simulink model "APP_VD"  (R2018a)
settings: configuration reference "cs_ert" (kept outside this file)
model workspace (MAT data in the model file):
  APP_VD_DT = 10
values from neighbouring files (symbols this model uses):
  APP_drLinRmp_C = 5.0    [APP_VD.sldd]
  APP_facLowNegPT1_C = 50.0    [APP_VD.sldd]
  APP_facLowPosPT1_C = 50.0    [APP_VD.sldd]
  APP_facMidNegPT1_C = 50.0    [APP_VD.sldd]
  APP_facMidPosPT1_C = 50.0    [APP_VD.sldd]
  APP_facUppNegPT1_C = 50.0    [APP_VD.sldd]
  APP_facUppPosPT1_C = 50.0    [APP_VD.sldd]
  APP_rThrFltLowNeg_C = 25.0    [APP_VD.sldd]
  APP_rThrFltLowPos_C = 25.0    [APP_VD.sldd]
  APP_rThrFltMidNeg_C = 50.0    [APP_VD.sldd]
  APP_rThrFltMidPos_C = 50.0    [APP_VD.sldd]
  APP_swtEnaFlt_C = 0    [APP_VD.sldd]
  APP_swtEnaUnJit_C = 0    [APP_VD.sldd]
  APP_uJitter_C = 3.0    [APP_VD.sldd]
  MoFAPP_rLinAPPCURCalMsgA_CUR : value not decoded    [APP_VD.sldd]
  MoFAPP_rLinAPPCURCalMsgA_CURX : value not decoded    [APP_VD.sldd]
  SigTst_rAPP_C = 0.0    [APP_VD.sldd]
  SigTst_swtAPP_C = 0    [APP_VD.sldd]
undefined symbols (not defined in the file or in its folder): Switch
libraries: sllib x2, simulink x1
settings Model: DataDictionary=APP_VD.sldd  Creator=zhoutinglin  LastModifiedBy=zhoutinglin

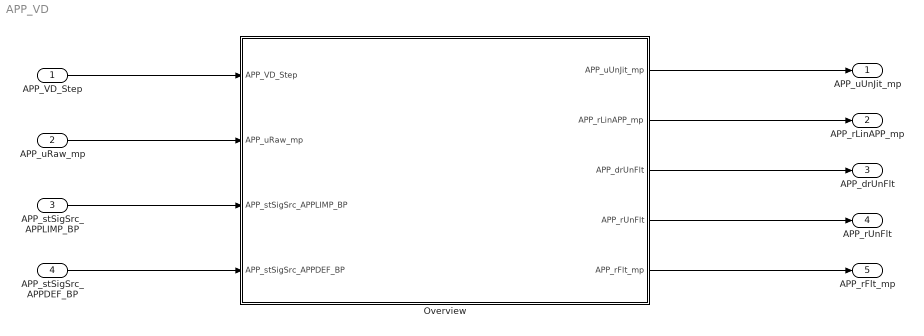
== system APP_VD ==
  APP_VD_Step : Inport  OutputFunctionCall=on
  APP_uRaw_mp : Inport  Description=Acceleration pedal position raw value  Port=2  OutMin=0  OutMax=5000  OutDataTypeStr=Volt_mV  Unit=mv  PortDimensions=[1 1]
  APP_stSigSrc_APPLIMP_BP : Inport  Description=Substitute operation active, accelerator pedal sensor value and accelerator pedal sensor increase are limited  Port=3  OutMin=0  OutMax=1  OutDataTypeStr=boolean  PortDimensions=[1 1]
  APP_stSigSrc_APPDEF_BP : Inport  Description=both the sensors are defective. Use the default value  Port=4  OutMin=0  OutMax=1  OutDataTypeStr=boolean  PortDimensions=[1 1]
  Overview : Subsystem
  APP_uUnJit_mp : Outport  Description=Acceleration pedal position unjittered value  OutMin=0  OutMax=5000  OutDataTypeStr=Volt_mV  Unit=mv  PortDimensions=[1 1]
  APP_rLinAPP_mp : Outport  Description=Linearisation ratio of accelerator pedal  Port=2  OutMin=0  OutMax=100  OutDataTypeStr=Percent  Unit=%  PortDimensions=[1 1]
  APP_drUnFlt : Outport  Description=Acceleration pedal position gradient of unfilterd value  Port=3  OutMin=-200  OutMax=200  OutDataTypeStr=Percent_s  Unit=%/ms  PortDimensions=[1 1]
  APP_rUnFlt : Outport  Description=Unfiltered APP value  Port=4  OutMin=0  OutMax=100  OutDataTypeStr=Percent  Unit=%  PortDimensions=[1 1]
  APP_rFlt_mp : Outport  Description=Acceleration pedal position filtered value  Port=5  OutMin=0  OutMax=100  OutDataTypeStr=Percent  Unit=%  PortDimensions=[1 1]
  wires:
  APP_VD_Step/1 -> Overview/1(APP_VD_Step)
  APP_uRaw_mp/1 -> Overview/2(APP_uRaw_mp)
  APP_stSigSrc_APPLIMP_BP/1 -> Overview/3(APP_stSigSrc_APPLIMP_BP)
  APP_stSigSrc_APPDEF_BP/1 -> Overview/4(APP_stSigSrc_APPDEF_BP)
  Overview/1(APP_uUnJit_mp) -> APP_uUnJit_mp/1
  Overview/2(APP_rLinAPP_mp) -> APP_rLinAPP_mp/1
  Overview/3(APP_drUnFlt) -> APP_drUnFlt/1
  Overview/4(APP_rUnFlt) -> APP_rUnFlt/1
  Overview/5(APP_rFlt_mp) -> APP_rFlt_mp/1

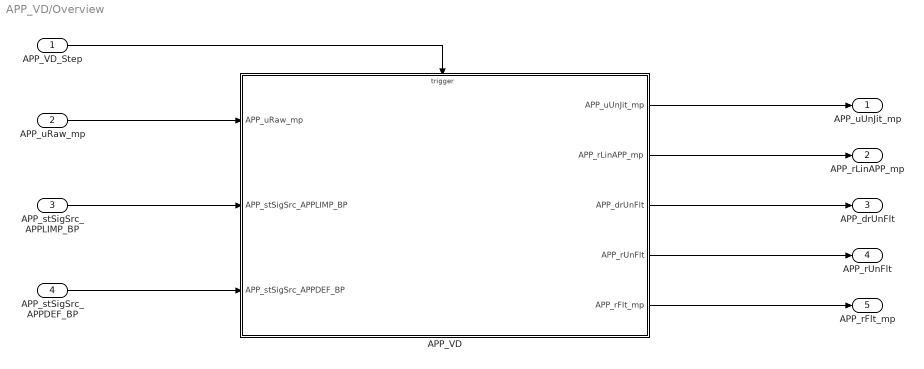
== system APP_VD/Overview ==
  APP_VD_Step : Inport
  APP_uRaw_mp : Inport  Port=2
  APP_stSigSrc_APPLIMP_BP : Inport  Port=3
  APP_stSigSrc_APPDEF_BP : Inport  Port=4
  APP_VD : Subsystem
  APP_uUnJit_mp : Outport
  APP_rLinAPP_mp : Outport  Port=2
  APP_drUnFlt : Outport  Port=3
  APP_rUnFlt : Outport  Port=4
  APP_rFlt_mp : Outport  Port=5
  wires:
  APP_uRaw_mp/1 -> APP_VD/1(APP_uRaw_mp)
  APP_stSigSrc_APPLIMP_BP/1 -> APP_VD/2(APP_stSigSrc_APPLIMP_BP)
  APP_stSigSrc_APPDEF_BP/1 -> APP_VD/3(APP_stSigSrc_APPDEF_BP)
  APP_VD/1(APP_uUnJit_mp) -> APP_uUnJit_mp/1
  APP_VD/2(APP_rLinAPP_mp) -> APP_rLinAPP_mp/1
  APP_VD/3(APP_drUnFlt) -> APP_drUnFlt/1
  APP_VD/4(APP_rUnFlt) -> APP_rUnFlt/1
  APP_VD/5(APP_rFlt_mp) -> APP_rFlt_mp/1
  APP_VD_Step/1 -> APP_VD/Trigger

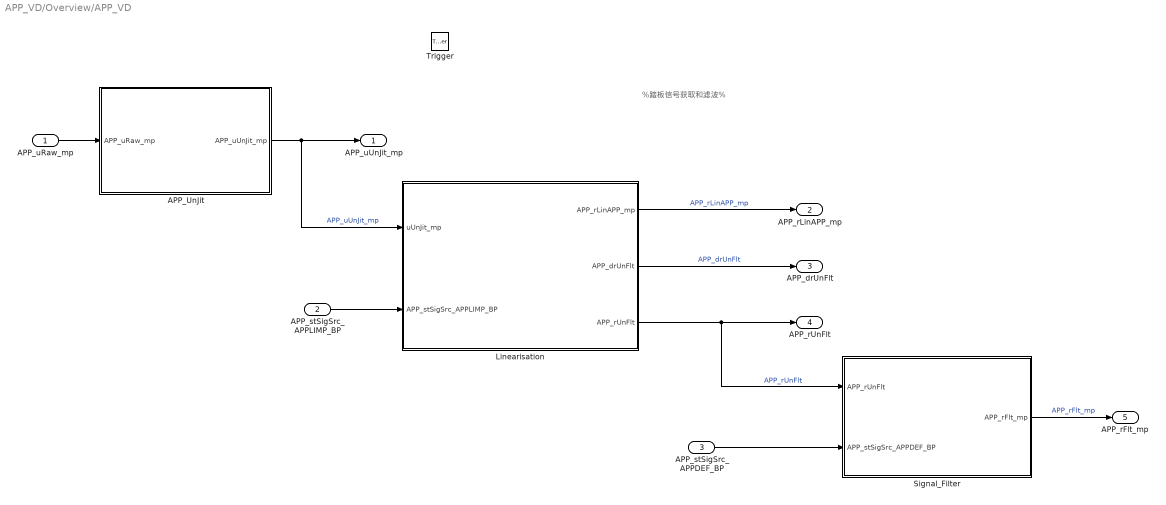
== system APP_VD/Overview/APP_VD ==
  note: %踏板信号获取和滤波%
  APP_uRaw_mp : Inport  Tag=mv
  APP_stSigSrc_APPLIMP_BP : Inport  Port=2
  APP_stSigSrc_APPDEF_BP : Inport  Port=3
  Trigger : TriggerPort  TriggerType=function-call  VariantControl=Variant  PortDimensions=1
  APP_UnJit : Subsystem
  Linearisation : Subsystem
  Signal_Filter : Subsystem
  APP_uUnJit_mp : Outport  Tag=mv
  APP_rLinAPP_mp : Outport  Tag=%  Port=2
  APP_drUnFlt : Outport  Tag=%/s  Port=3
  APP_rUnFlt : Outport  Tag=%  Port=4
  APP_rFlt_mp : Outport  Tag=%  Port=5
  wires:
  APP_uRaw_mp/1 -> APP_UnJit/1(APP_uRaw_mp)
  Signal_Filter/1(APP_rFlt_mp) -> APP_rFlt_mp/1  "APP_rFlt_mp"
  Linearisation/2(APP_drUnFlt) -> APP_drUnFlt/1  "APP_drUnFlt"
  APP_stSigSrc_APPDEF_BP/1 -> Signal_Filter/2(APP_stSigSrc_APPDEF_BP)
  Linearisation/3(APP_rUnFlt) -> APP_rUnFlt/1, Signal_Filter/1(APP_rUnFlt)  "APP_rUnFlt"
  Linearisation/1(APP_rLinAPP_mp) -> APP_rLinAPP_mp/1  "APP_rLinAPP_mp"
  APP_stSigSrc_APPLIMP_BP/1 -> Linearisation/2(APP_stSigSrc_APPLIMP_BP)
  APP_UnJit/1(APP_uUnJit_mp) -> APP_uUnJit_mp/1, Linearisation/1(uUnJit_mp)  "APP_uUnJit_mp"

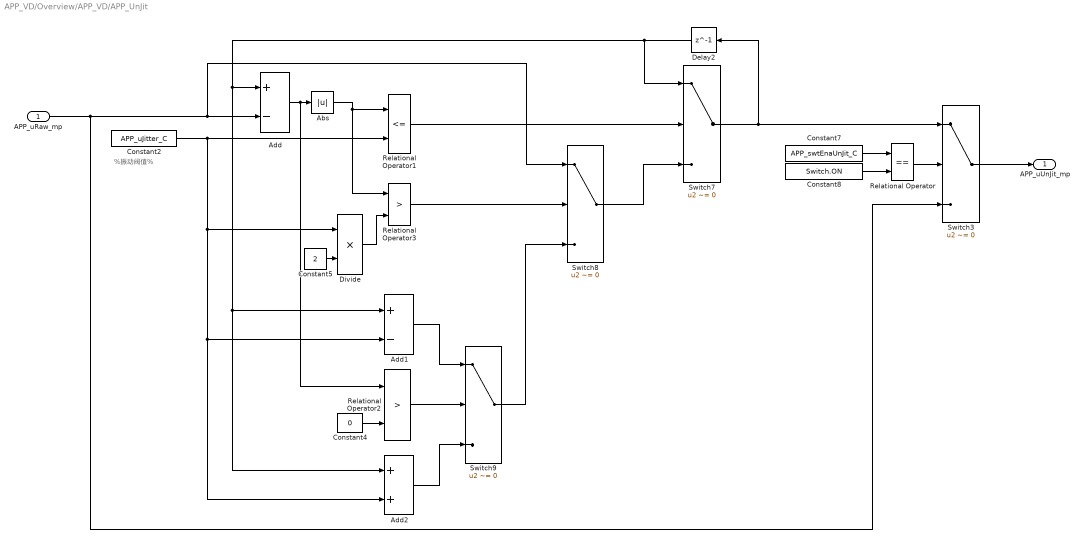
== system APP_VD/Overview/APP_VD/APP_UnJit ==
  note: %振动阀值%
  APP_uRaw_mp : Inport
  Abs : Abs  OutDataTypeStr=Inherit: Inherit via back propagation
  Add : Sum  Inputs=+-  InputSameDT=on
  Add1 : Sum  Inputs=+-  InputSameDT=on
  Add2 : Sum  InputSameDT=on
  Constant2 : Constant  Value=APP_uJitter_C
  Constant4 : Constant  Value=0  OutDataTypeStr=Inherit: Inherit via back propagation
  Constant5 : Constant  Value=2  OutDataTypeStr=Inherit: Inherit via back propagation
  Constant7 : Constant  Value=APP_swtEnaUnJit_C
  Constant8 : Constant  Value=Switch.ON  OutDataTypeStr=Inherit: Inherit via back propagation
  Delay2 : Delay  DelayLength=1  InitialCondition=0
  Divide : Product  Inputs=**  OutDataTypeStr=Inherit: Inherit via back propagation
  Relational Operator : RelationalOperator  Operator===  OutDataTypeStr=boolean  RndMeth=Simplest  InputSameDT=on
  Relational Operator1 : RelationalOperator  Operator=<=  OutDataTypeStr=boolean  RndMeth=Nearest  InputSameDT=on
  Relational Operator2 : RelationalOperator  Operator=>  OutDataTypeStr=boolean  RndMeth=Nearest  InputSameDT=on
  Relational Operator3 : RelationalOperator  Operator=>  OutDataTypeStr=boolean  RndMeth=Nearest  InputSameDT=on
  Switch{3,7..9} (4 alike) : Switch  Criteria=u2 ~= 0  InputSameDT=on
  APP_uUnJit_mp : Outport
  wires:
  Constant2/1 -> Add2/2, Add1/2, Divide/1, Relational Operator1/2
  Relational Operator/1 -> Switch3/2
  Add1/1 -> Switch9/1
  Add2/1 -> Switch9/3
  Add/1 -> Abs/1, Relational Operator2/1
  Abs/1 -> Relational Operator1/1, Relational Operator3/1
  Constant8/1 -> Relational Operator/2
  Switch9/1 -> Switch8/3
  Divide/1 -> Relational Operator3/2
  Relational Operator1/1 -> Switch7/2
  Relational Operator3/1 -> Switch8/2
  Delay2/1 -> Add1/1, Add2/1, Add/1, Switch7/1
  Switch7/1 -> Switch3/1, Delay2/1
  Constant5/1 -> Divide/2
  APP_uRaw_mp/1 -> Switch3/3, Add/2, Switch8/1
  Relational Operator2/1 -> Switch9/2
  Constant4/1 -> Relational Operator2/2
  Switch8/1 -> Switch7/3
  Constant7/1 -> Relational Operator/1
  Switch3/1 -> APP_uUnJit_mp/1

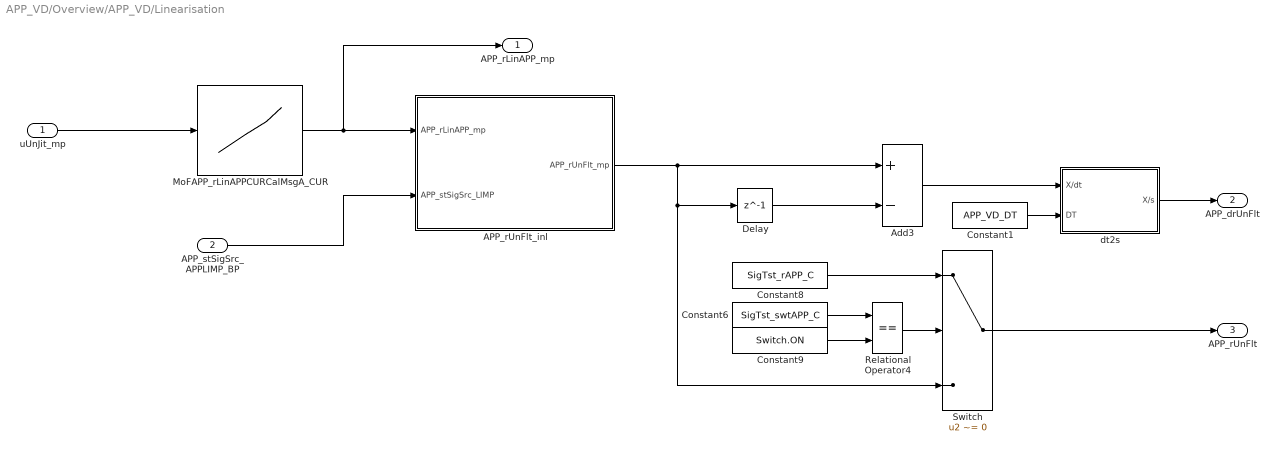
== system APP_VD/Overview/APP_VD/Linearisation ==
  uUnJit_mp : Inport
  APP_stSigSrc_APPLIMP_BP : Inport  Tag=-  Port=2
  APP_rUnFlt_inl : Subsystem
  Add3 : Sum  Inputs=+-  InputSameDT=on
  Constant1 : Constant  Value=APP_VD_DT  OutDataTypeStr=Inherit: Inherit via back propagation
  Constant6 : Constant  Value=SigTst_swtAPP_C
  Constant8 : Constant  Value=SigTst_rAPP_C
  Constant9 : Constant  Value=Switch.ON  OutDataTypeStr=Inherit: Inherit via back propagation
  Delay : Delay  DelayLength=1  InitialCondition=0
  MoFAPP_rLinAPPCURCalMsgA_CUR : Lookup_n-D  NumberOfTableDimensions=1  BreakpointsForDimension1=MoFAPP_rLinAPPCURCalMsgA_CURX  IndexSearchMethod=Linear search  BeginIndexSearchUsingPreviousIndexResult=on  UseOneInputPortForAllInputData=on  Table=MoFAPP_rLinAPPCURCalMsgA_CUR  ExtrapMethod=Clip  UseLastTableValue=on  InternalRulePriority=Speed  OutDataTypeStr=Inherit: Inherit via back propagation  SaturateOnIntegerOverflow=on
  Relational Operator4 : RelationalOperator  Operator===  OutDataTypeStr=boolean  RndMeth=Simplest  InputSameDT=on
  Switch : Switch  Criteria=u2 ~= 0  InputSameDT=on
  dt2s : Subsystem
  APP_rLinAPP_mp : Outport  Tag=%%
  APP_drUnFlt : Outport  Tag=%%  Port=2
  APP_rUnFlt : Outport  Tag=%%  Port=3
  wires:
  APP_stSigSrc_APPLIMP_BP/1 -> APP_rUnFlt_inl/2(APP_stSigSrc_LIMP)
  uUnJit_mp/1 -> MoFAPP_rLinAPPCURCalMsgA_CUR/1
  Relational Operator4/1 -> Switch/2
  Constant6/1 -> Relational Operator4/1
  Constant9/1 -> Relational Operator4/2
  Constant8/1 -> Switch/1
  Switch/1 -> APP_rUnFlt/1
  Delay/1 -> Add3/2
  APP_rUnFlt_inl/1(APP_rUnFlt_mp) -> Switch/3, Delay/1, Add3/1
  MoFAPP_rLinAPPCURCalMsgA_CUR/1 -> APP_rLinAPP_mp/1, APP_rUnFlt_inl/1(APP_rLinAPP_mp)
  Constant1/1 -> dt2s/2(DT)
  Add3/1 -> dt2s/1(X/dt)
  dt2s/1(X/s) -> APP_drUnFlt/1

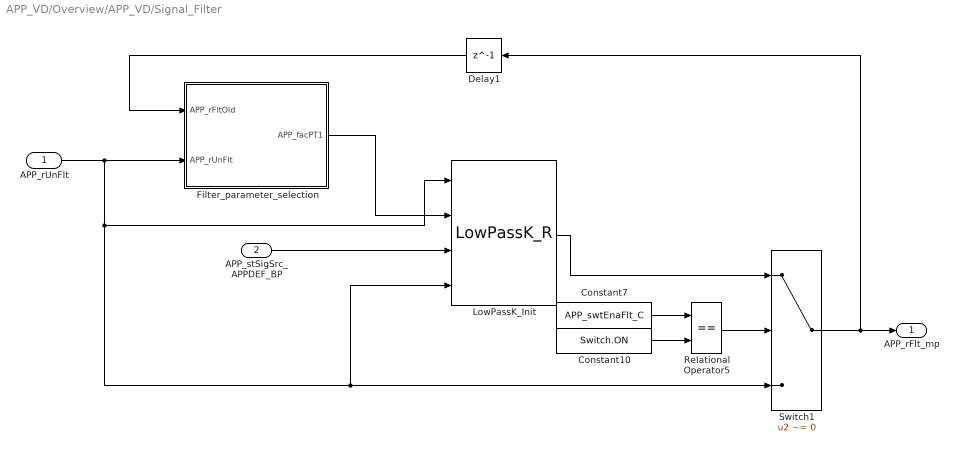
== system APP_VD/Overview/APP_VD/Signal_Filter ==
  APP_rUnFlt : Inport
  APP_stSigSrc_APPDEF_BP : Inport  Tag=-  Port=2
  Constant10 : Constant  Value=Switch.ON  OutDataTypeStr=Inherit: Inherit via back propagation
  Constant7 : Constant  Value=APP_swtEnaFlt_C
  Delay1 : Delay  DelayLength=1  InitialCondition=0
  Filter_parameter_selection : Subsystem  TreatAsAtomicUnit=on
  LowPassK_Init : sllib/LowPassK_R
      settings: SourceProductName=sllib
  Relational Operator5 : RelationalOperator  Operator===  OutDataTypeStr=boolean  RndMeth=Simplest  InputSameDT=on
  Switch1 : Switch  Criteria=u2 ~= 0  InputSameDT=on
  APP_rFlt_mp : Outport  Tag=%%
  wires:
  Relational Operator5/1 -> Switch1/2
  Constant10/1 -> Relational Operator5/2
  Constant7/1 -> Relational Operator5/1
  LowPassK_Init/1 -> Switch1/1
  Filter_parameter_selection/1(APP_facPT1) -> LowPassK_Init/2
  Switch1/1 -> APP_rFlt_mp/1, Delay1/1
  Delay1/1 -> Filter_parameter_selection/1(APP_rFltOld)
  APP_rUnFlt/1 -> LowPassK_Init/4, Switch1/3, LowPassK_Init/1, Filter_parameter_selection/2(APP_rUnFlt)
  APP_stSigSrc_APPDEF_BP/1 -> LowPassK_Init/3

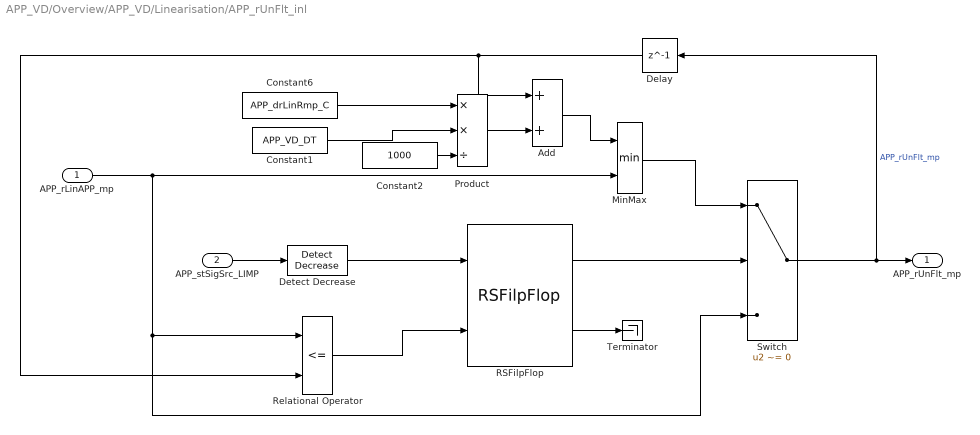
== system APP_VD/Overview/APP_VD/Linearisation/APP_rUnFlt_inl ==
  APP_rLinAPP_mp : Inport
  APP_stSigSrc_LIMP : Inport  Port=2
  Add : Sum  InputSameDT=on
  Constant1 : Constant  Value=APP_VD_DT  OutDataTypeStr=Inherit: Inherit via back propagation
  Constant2 : Constant  Value=1000  OutDataTypeStr=int16
  Constant6 : Constant  Value=APP_drLinRmp_C
  Delay : Delay  DelayLength=1  InitialCondition=0
  Detect Decrease : simulink/Logic and Bit Operations/Detect Decrease  vinit=0.0  OutDataTypeStr=boolean
  MinMax : MinMax  Inputs=2
  Product : Product  Inputs=**/  OutDataTypeStr=Inherit: Inherit via back propagation
  RSFilpFlop : sllib/RSFilpFlop
      settings: SourceProductName=sllib
  Relational Operator : RelationalOperator  Operator=<=  OutDataTypeStr=boolean  RndMeth=Simplest
  Switch : Switch  Criteria=u2 ~= 0  InputSameDT=on
  Terminator : Terminator
  APP_rUnFlt_mp : Outport
  wires:
  RSFilpFlop/2 -> Terminator/1
  Relational Operator/1 -> RSFilpFlop/2
  APP_stSigSrc_LIMP/1 -> Detect Decrease/1
  Detect Decrease/1 -> RSFilpFlop/1
  Delay/1 -> Relational Operator/2, Add/1
  Switch/1 -> APP_rUnFlt_mp/1, Delay/1  "APP_rUnFlt_mp"
  Add/1 -> MinMax/1
  APP_rLinAPP_mp/1 -> MinMax/2, Switch/3, Relational Operator/1
  MinMax/1 -> Switch/1
  RSFilpFlop/1 -> Switch/2
  Product/1 -> Add/2
  Constant6/1 -> Product/1
  Constant1/1 -> Product/2
  Constant2/1 -> Product/3

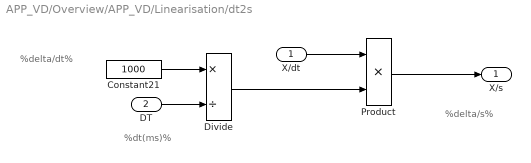
== system APP_VD/Overview/APP_VD/Linearisation/dt2s ==
  note: %delta/s%
  note: %delta/dt%
  note: %dt(ms)%
  X/dt : Inport
  DT : Inport  Port=2
  Constant21 : Constant  Value=1000  OutDataTypeStr=int16
  Divide : Product  Inputs=*/  OutDataTypeStr=int16  RndMeth=Round  SaturateOnIntegerOverflow=on
  Product : Product  OutDataTypeStr=Inherit: Inherit via back propagation  RndMeth=Round  SaturateOnIntegerOverflow=on
  X/s : Outport
  wires:
  Product/1 -> X/s/1
  X/dt/1 -> Product/1
  Constant21/1 -> Divide/1
  Divide/1 -> Product/2
  DT/1 -> Divide/2

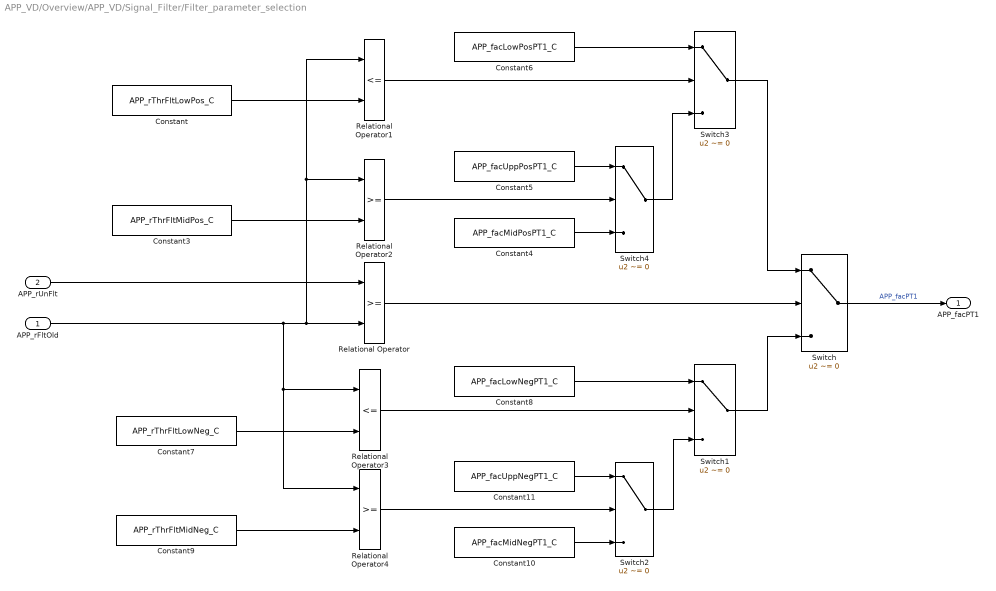
== system APP_VD/Overview/APP_VD/Signal_Filter/Filter_parameter_selection ==
  APP_rFltOld : Inport
  APP_rUnFlt : Inport  Port=2
  Constant : Constant  Value=APP_rThrFltLowPos_C
  Constant10 : Constant  Value=APP_facMidNegPT1_C
  Constant11 : Constant  Value=APP_facUppNegPT1_C
  Constant3 : Constant  Value=APP_rThrFltMidPos_C
  Constant4 : Constant  Value=APP_facMidPosPT1_C
  Constant5 : Constant  Value=APP_facUppPosPT1_C
  Constant6 : Constant  Value=APP_facLowPosPT1_C
  Constant7 : Constant  Value=APP_rThrFltLowNeg_C
  Constant8 : Constant  Value=APP_facLowNegPT1_C
  Constant9 : Constant  Value=APP_rThrFltMidNeg_C
  Relational Operator : RelationalOperator  OutDataTypeStr=boolean  RndMeth=Nearest
  Relational Operator1 : RelationalOperator  Operator=<=  OutDataTypeStr=boolean  RndMeth=Nearest
  Relational Operator2 : RelationalOperator  OutDataTypeStr=boolean  RndMeth=Nearest
  Relational Operator3 : RelationalOperator  Operator=<=  OutDataTypeStr=boolean  RndMeth=Nearest
  Relational Operator4 : RelationalOperator  OutDataTypeStr=boolean  RndMeth=Nearest
  Switch{,1..4} (5 alike) : Switch  Criteria=u2 ~= 0  Threshold=1  InputSameDT=on
  APP_facPT1 : Outport
  wires:
  Constant/1 -> Relational Operator1/2
  Constant3/1 -> Relational Operator2/2
  Constant7/1 -> Relational Operator3/2
  Constant9/1 -> Relational Operator4/2
  Relational Operator/1 -> Switch/2
  Constant8/1 -> Switch1/1
  Constant11/1 -> Switch2/1
  Constant10/1 -> Switch2/3
  Relational Operator4/1 -> Switch2/2
  Switch2/1 -> Switch1/3
  Relational Operator3/1 -> Switch1/2
  Constant6/1 -> Switch3/1
  Switch4/1 -> Switch3/3
  Constant5/1 -> Switch4/1
  Constant4/1 -> Switch4/3
  Relational Operator2/1 -> Switch4/2
  Switch3/1 -> Switch/1
  Relational Operator1/1 -> Switch3/2
  APP_rFltOld/1 -> Relational Operator2/1, Relational Operator1/1, Relational Operator/2, Relational Operator3/1, Relational Operator4/1
  APP_rUnFlt/1 -> Relational Operator/1
  Switch1/1 -> Switch/3
  Switch/1 -> APP_facPT1/1  "APP_facPT1"
